simulink model "Neurofeedback_GetConnectivity_IncrementalAvg"  (R2021b)
settings: Solver=ode23tb  StartTime=0.0  StopTime=130  FixedStep=1  RelTol=1e-3
libraries: simulink x6
settings Model: SnapshotBufferSize=100  SnapshotInterval=100  Creator=mariodelossantos  LastModifiedBy=mdls3

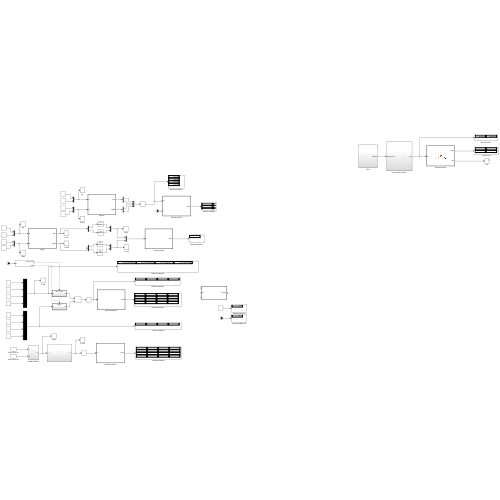
[thumbnail: Simulink's stored preview of the top-level diagram]
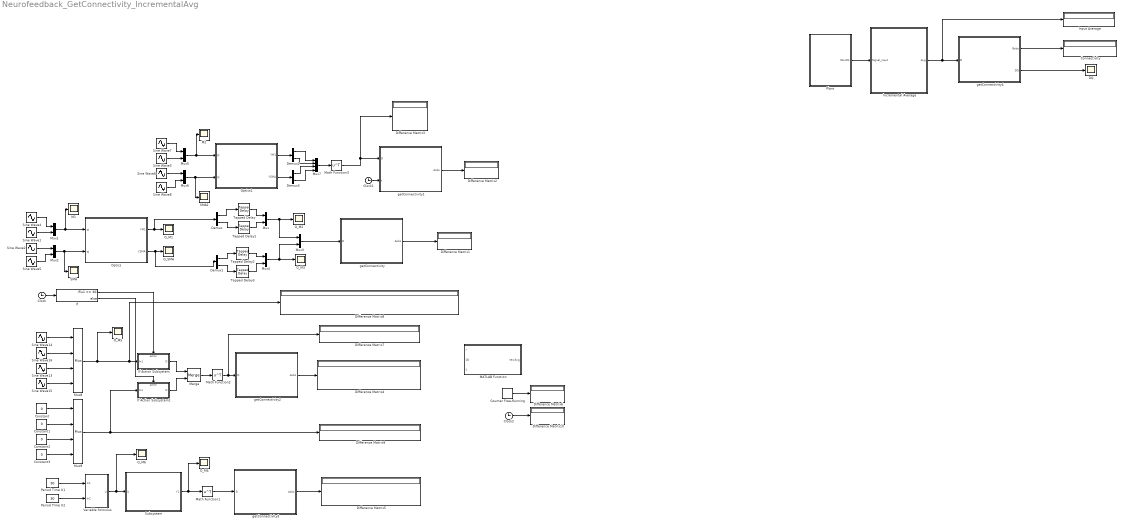
== system Neurofeedback_GetConnectivity_IncrementalAvg ==
  Clock : Clock
  Clock1 : Clock
  Clock2 : Clock
  Connectivity : Display
  Constant{,1..3} (4 alike) : Constant  Value=0
  Counter Free-Running : simulink/Sources/Counter Free-Running  NumBits=16  tsamp=-1
  DQ : Scope
  Demux{,1..3} (4 alike) : Demux  Outputs=2
  Difference Matrix{1..10} (10 alike) : Display
  If : If  IfExpression=u1 == 30
  If Action Subsystem : Subsystem  TreatAsAtomicUnit=on
  If Action Subsystem1 : Subsystem  TreatAsAtomicUnit=on
  Incremental Average : Subsystem
  "Input Average " : Display
  M1 : Scope
  M2 : Scope
  MATLAB Function : MATLAB Function  TreatAsAtomicUnit=on
  Math Function1 : Math  Operator=transpose  SaturateOnIntegerOverflow=on
  Math Function2 : Math  Operator=transpose  SaturateOnIntegerOverflow=on
  Math Function3 : Math  Operator=transpose  SaturateOnIntegerOverflow=on
  Merge : Merge  InitialOutput=[0 0 0 0]
  Mux{,1..6} (7 alike) : Mux  Inputs=2
  Mux7 : Mux
  Mux8 : Mux
  Mux9 : Mux
  O_M{1..6} (6 alike) : Scope
  O_SMA : Scope
  Optics : MATLAB Function  TreatAsAtomicUnit=on
  Optics1 : MATLAB Function  TreatAsAtomicUnit=on
  Period Time U1 : Constant  Value=30
  Period Time U2 : Constant  Value=30
  Plant : Subsystem
  SMA : Scope
  SMA1 : Scope
  Sine Wave1 : Sin  Amplitude=1.2  Frequency=0.8  SampleTime=0
  Sine Wave13 : Sin  Amplitude=0.8  Frequency=0.6  SampleTime=0
  Sine Wave14 : Sin  Frequency=0.9  SampleTime=0
  Sine Wave15 : Sin  Frequency=0.4  SampleTime=0
  Sine Wave16 : Sin  Amplitude=1.2  Frequency=0.8  SampleTime=0
  Sine Wave2 : Sin  Amplitude=0.8  Frequency=0.8  SampleTime=0
  Sine Wave3 : Sin  Amplitude=1.2  Frequency=0.8  SampleTime=0
  Sine Wave{4..5,7..8} (4 alike) : Sin  Frequency=0.8  SampleTime=0
  Sine Wave6 : Sin  Amplitude=0.8  Frequency=0.8  SampleTime=0
  Subsystem : Subsystem
  Tapped Delay{,1..3} (4 alike) : simulink/Discrete/Tapped Delay  vinit=0.0  samptime=-1  NumDelays=29  DelayOrder=Oldest  includeCurrent=on
  Variable Stimulus : Subsystem
  getConnectivity : MATLAB Function  TreatAsAtomicUnit=on  SystemSampleTime=0
  getConnectivity1 : MATLAB Function  TreatAsAtomicUnit=on  SystemSampleTime=0
  getConnectivity2 : MATLAB Function  TreatAsAtomicUnit=on  SystemSampleTime=0
  getConnectivity3 : MATLAB Function  TreatAsAtomicUnit=on  SystemSampleTime=0
  getConnectivity4 : MATLAB Function  TreatAsAtomicUnit=on  SystemSampleTime=0
  wires:
  getConnectivity/1(Aobs) -> Difference Matrix1/1
  Sine Wave4/1 -> Mux1/1
  Sine Wave5/1 -> Mux2/2
  Sine Wave1/1 -> Mux1/2
  Sine Wave2/1 -> Mux2/1
  Optics/1(YM1) -> O_M1/1, Demux/1
  Optics/2(YSMA) -> Demux1/1, O_SMA/1
  Mux2/1 -> SMA/1, Optics/2(qj)
  Mux1/1 -> M1/1, Optics/1(pj)
  Demux/1 -> Tapped Delay/1
  Demux/2 -> Tapped Delay1/1
  Tapped Delay/1 -> Mux/1
  Tapped Delay1/1 -> Mux/2
  Mux/1 -> O_M2/1, Mux3/1
  Mux3/1 -> getConnectivity/1(D)
  Mux4/1 -> O_M3/1, Mux3/2
  Clock/1 -> If/1
  If/1 -> If Action Subsystem/Action
  Tapped Delay2/1 -> Mux4/1
  Demux1/1 -> Tapped Delay2/1
  Demux1/2 -> Tapped Delay3/1
  Tapped Delay3/1 -> Mux4/2
  If/2 -> If Action Subsystem1/Action
  If Action Subsystem/1(D) -> Merge/1
  If Action Subsystem1/1(D) -> Merge/2
  Demux3/1 -> Mux7/3
  Clock1/1 -> getConnectivity1/2(t)
  Demux3/2 -> Mux7/4
  Mux6/1 -> SMA1/1, Optics1/2(qj)
  Sine Wave8/1 -> Mux6/2
  Demux2/1 -> Mux7/1
  Optics1/2(YSMA) -> Demux3/1
  Sine Wave7/1 -> Mux5/1
  Mux5/1 -> M2/1, Optics1/1(pj)
  Optics1/1(YM1) -> Demux2/1
  Sine Wave6/1 -> Mux6/1
  Sine Wave3/1 -> Mux5/2
  Demux2/2 -> Mux7/2
  getConnectivity1/1(Aobs) -> Difference Matrix2/1
  getConnectivity2/1(Aobs) -> Difference Matrix4/1
  getConnectivity3/1(Aobs) -> Difference Matrix5/1
  Merge/1 -> Math Function2/1
  Math Function1/1 -> getConnectivity3/1(D)
  Mux8/1 -> O_M5/1, Difference Matrix8/1, If Action Subsystem/1(In1)
  Sine Wave13/1 -> Mux8/3
  Sine Wave16/1 -> Mux8/2
  Sine Wave15/1 -> Mux8/4
  Sine Wave14/1 -> Mux8/1
  Mux9/1 -> If Action Subsystem1/1(In1), Difference Matrix9/1
  Constant/1 -> Mux9/1
  Constant1/1 -> Mux9/2
  Constant2/1 -> Mux9/3
  Constant3/1 -> Mux9/4
  Math Function2/1 -> getConnectivity2/1(D), Difference Matrix7/1
  Subsystem/1(Y1) -> O_M4/1, Math Function1/1
  Period Time U1/1 -> Variable Stimulus/1(In1)
  Period Time U2/1 -> Variable Stimulus/2(In2)
  Variable Stimulus/1(U) -> O_M6/1, Subsystem/1(U)
  Mux7/1 -> Math Function3/1
  Math Function3/1 -> Difference Matrix3/1, getConnectivity1/1(D)
  Counter Free-Running/1 -> Difference Matrix6/1
  Clock2/1 -> Difference Matrix10/1
  getConnectivity4/1(Bobs) -> Connectivity/1
  Incremental Average/1(Avg) -> getConnectivity4/1(D), "Input Average "/1
  getConnectivity4/2(DQ) -> DQ/1
  Plant/1(DH-DQ) -> Incremental Average/1(Signal_input)

== system Neurofeedback_GetConnectivity_IncrementalAvg/If Action Subsystem ==
  In1 : Inport
  Action Port : ActionPort  ActionPortLabel=if(u1 == 30)
  D : Outport
  wires:
  In1/1 -> D/1

== system Neurofeedback_GetConnectivity_IncrementalAvg/If Action Subsystem1 ==
  In1 : Inport
  Action Port : ActionPort  ActionPortLabel=else
  D : Outport
  wires:
  In1/1 -> D/1

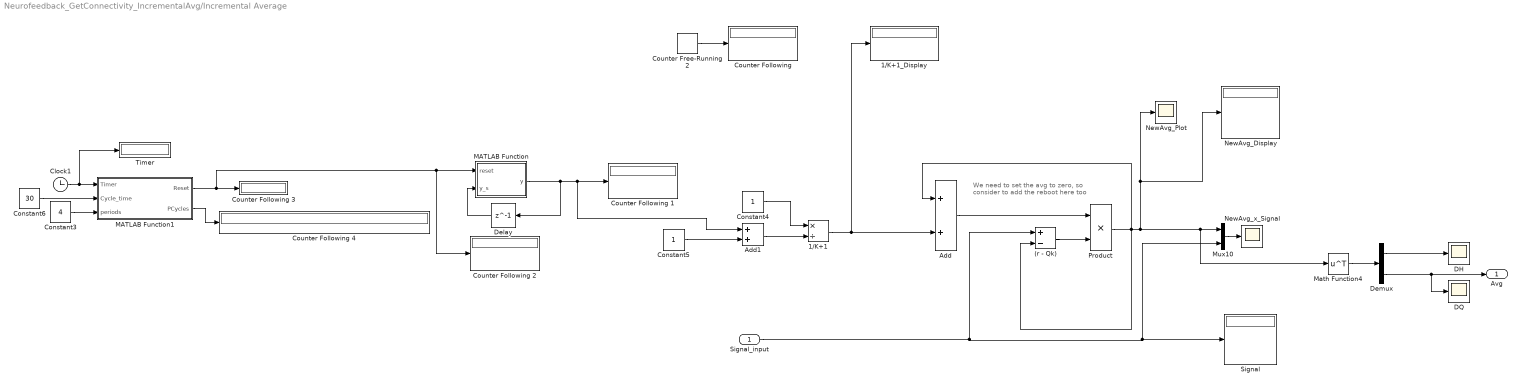
== system Neurofeedback_GetConnectivity_IncrementalAvg/Incremental Average ==
  note: We need to set the avg to zero, so consider to add the reboot here too
  Signal_input : Inport
  (r - Qk) : Sum  Inputs=+-
  1/K+1 : Product  Inputs=*/
  1/K+1_Display : Display
  Add : Sum
  Add1 : Sum
  Clock1 : Clock
  Constant3 : Constant  Value=4
  Constant4 : Constant
  Constant5 : Constant
  Constant6 : Constant  Value=30
  Counter Free-Running2 : simulink/Sources/Counter Free-Running  NumBits=16  tsamp=-1
  Counter Following {,1..4} (5 alike) : Display
  DH : Scope
  DQ : Scope
  Delay : Delay  DelayLength=1  InitialCondition=0
  Demux : Demux  Outputs=2
  MATLAB Function : MATLAB Function  TreatAsAtomicUnit=on
  MATLAB Function1 : MATLAB Function  TreatAsAtomicUnit=on
  Math Function4 : Math  Operator=transpose  SaturateOnIntegerOverflow=on
  Mux10 : Mux  Inputs=2
  NewAvg_Display : Display
  NewAvg_Plot : Scope
  NewAvg_x_Signal : Scope
  Product : Product
  Signal : Display
  Timer : Display
  Avg : Outport
  wires:
  (r - Qk)/1 -> Product/2
  Signal_input/1 -> Signal/1, Mux10/2, (r - Qk)/1
  Add/1 -> Product/1
  Mux10/1 -> NewAvg_x_Signal/1
  Product/1 -> Add/1, (r - Qk)/2, NewAvg_Plot/1, NewAvg_Display/1, Math Function4/1, Mux10/1
  Math Function4/1 -> Demux/1
  Demux/2 -> Avg/1, DQ/1
  Demux/1 -> DH/1
  Constant4/1 -> 1/K+1/1
  Counter Free-Running2/1 -> "Counter Following "/1
  Constant5/1 -> Add1/2
  Add1/1 -> 1/K+1/2
  1/K+1/1 -> 1/K+1_Display/1, Add/2
  MATLAB Function/1(y) -> Add1/1, Counter Following 1/1, Delay/1
  Delay/1 -> MATLAB Function/2(y_s)
  MATLAB Function1/1(Reset) -> Counter Following 2/1, MATLAB Function/1(reset), Counter Following 3/1
  MATLAB Function1/2(PCycles) -> Counter Following 4/1
  Constant6/1 -> MATLAB Function1/2(Cycle_time)
  Constant3/1 -> MATLAB Function1/3(periods)
  Clock1/1 -> MATLAB Function1/1(Timer), Timer/1

== system Neurofeedback_GetConnectivity_IncrementalAvg/Plant ==
  Human Agent : Subsystem
  Period Time U3 : Constant  Value=30
  Period Time U4 : Constant  Value=30
  Stimulus : Scope
  Variable Stimulus1 : Subsystem
  fNIRS : Scope
  DH-DQ : Outport
  wires:
  Human Agent/1(fNIRS) -> fNIRS/1
  Period Time U3/1 -> Variable Stimulus1/1(In1)
  Period Time U4/1 -> Variable Stimulus1/2(In2)
  Human Agent/2(DH-DQ) -> DH-DQ/1
  Variable Stimulus1/1(U) -> Stimulus/1, Human Agent/1(Stimulus)

== system Neurofeedback_GetConnectivity_IncrementalAvg/Subsystem ==
  U : Inport
  Deltas-Hemo1 : Subsystem
  Hemodynamics1 : Subsystem
  Neurodynamics1 : Subsystem
  Optics2 : Subsystem
  Z : Scope
  y1 : Scope
  Y1 : Outport
  wires:
  Deltas-Hemo1/1(DH) -> Optics2/1(DH)
  U/1 -> Neurodynamics1/1(U)
  Neurodynamics1/1(Z) -> Z/1, Hemodynamics1/1(Zj)  "Zj"
  Deltas-Hemo1/2(DQ) -> Optics2/2(DQ)
  Optics2/1(Y1) -> y1/1, Y1/1
  Hemodynamics1/1(Pj) -> Deltas-Hemo1/1(pj)
  Hemodynamics1/2(qj) -> Deltas-Hemo1/2(qj)

== system Neurofeedback_GetConnectivity_IncrementalAvg/Variable Stimulus ==
  In1 : Inport
  In2 : Inport  Port=2
  Duty-Cycle-U1 : Constant  Value=0.16667  OutMin=[0]  OutMax=[0.8]
  Duty-Cycle-U2 : Constant  Value=0.16667  OutMin=[0]  OutMax=[0.8]
  Mux : Mux  Inputs=2
  Variable Pulse Generator1 : VariablePulseGenerator  RunAtFixedTimeIntervals=on
  Variable Pulse Generator2 : VariablePulseGenerator  RunAtFixedTimeIntervals=on
  U : Outport
  wires:
  In2/1 -> Variable Pulse Generator1/2
  Mux/1 -> U/1
  Variable Pulse Generator1/1 -> Mux/2
  Duty-Cycle-U2/1 -> Variable Pulse Generator1/1
  In1/1 -> Variable Pulse Generator2/2
  Duty-Cycle-U1/1 -> Variable Pulse Generator2/1
  Variable Pulse Generator2/1 -> Mux/1

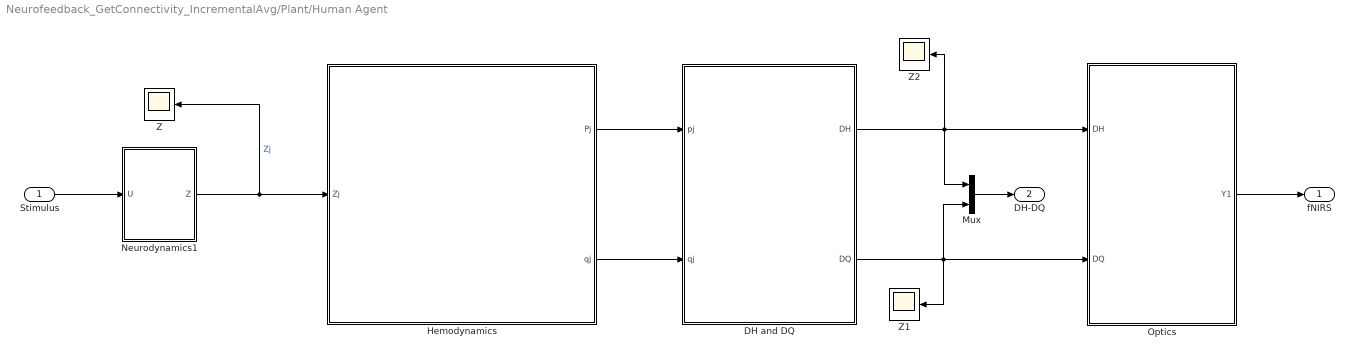
== system Neurofeedback_GetConnectivity_IncrementalAvg/Plant/Human Agent ==
  Stimulus : Inport
  DH and DQ : Subsystem
  Hemodynamics : Subsystem
  Mux : Mux  Inputs=2
  Neurodynamics1 : Subsystem
  Optics : Subsystem
  Z : Scope
  Z1 : Scope
  Z2 : Scope
  fNIRS : Outport
  DH-DQ : Outport  Port=2
  wires:
  Hemodynamics/1(Pj) -> DH and DQ/1(pj)
  Hemodynamics/2(qj) -> DH and DQ/2(qj)
  Neurodynamics1/1(Z) -> Z/1, Hemodynamics/1(Zj)  "Zj"
  Stimulus/1 -> Neurodynamics1/1(U)
  DH and DQ/1(DH) -> Z2/1, Mux/1, Optics/1(DH)
  DH and DQ/2(DQ) -> Z1/1, Mux/2, Optics/2(DQ)
  Optics/1(Y1) -> fNIRS/1
  Mux/1 -> DH-DQ/1

== system Neurofeedback_GetConnectivity_IncrementalAvg/Plant/Variable Stimulus1 ==
  In1 : Inport
  In2 : Inport  Port=2
  Duty-Cycle-U1 : Constant  Value=0.16667  OutMin=[0]  OutMax=[0.8]
  Duty-Cycle-U2 : Constant  Value=0.16667  OutMin=[0]  OutMax=[0.8]
  Mux : Mux  Inputs=2
  Variable Pulse Generator1 : VariablePulseGenerator  RunAtFixedTimeIntervals=on  SampleTime=1/100
  Variable Pulse Generator2 : VariablePulseGenerator  RunAtFixedTimeIntervals=on  SampleTime=1/100
  U : Outport
  wires:
  In2/1 -> Variable Pulse Generator1/2
  Mux/1 -> U/1
  Variable Pulse Generator1/1 -> Mux/2
  Duty-Cycle-U2/1 -> Variable Pulse Generator1/1
  In1/1 -> Variable Pulse Generator2/2
  Duty-Cycle-U1/1 -> Variable Pulse Generator2/1
  Variable Pulse Generator2/1 -> Mux/1

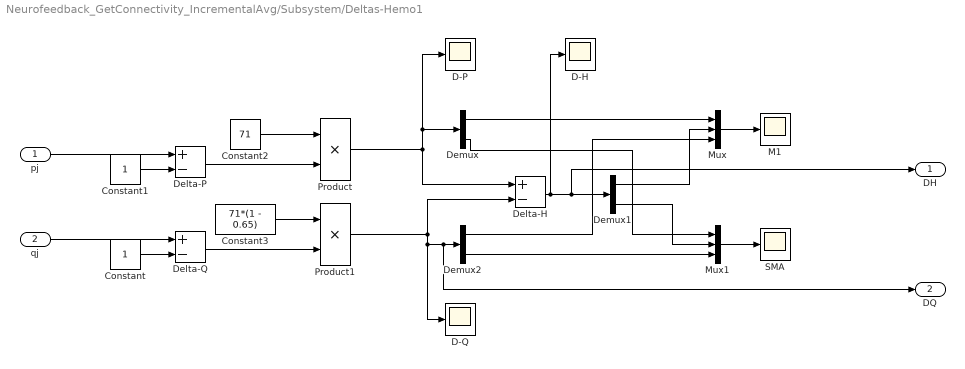
== system Neurofeedback_GetConnectivity_IncrementalAvg/Subsystem/Deltas-Hemo1 ==
  pj : Inport
  qj : Inport  Port=2
  Constant : Constant
  Constant1 : Constant
  Constant2 : Constant  Value=71
  Constant3 : Constant  Value=71*(1 - 0.65)
  D-H : Scope
  D-P : Scope
  D-Q : Scope
  Delta-H : Sum  Inputs=+-
  Delta-P : Sum  Inputs=+-
  Delta-Q : Sum  Inputs=+-
  Demux : Demux  Outputs=2
  Demux1 : Demux  Outputs=2
  Demux2 : Demux  Outputs=2
  M1 : Scope
  Mux : Mux  Inputs=3
  Mux1 : Mux  Inputs=3
  Product : Product
  Product1 : Product
  SMA : Scope
  DH : Outport
  DQ : Outport  Port=2
  wires:
  Constant2/1 -> Product/1
  Delta-Q/1 -> Product1/2
  Constant3/1 -> Product1/1
  Demux2/2 -> Mux1/3
  pj/1 -> Delta-P/1
  Mux1/1 -> SMA/1
  Demux/2 -> Mux1/1
  Mux/1 -> M1/1
  Constant/1 -> Delta-Q/2
  Delta-P/1 -> Product/2
  Product1/1 -> DQ/1, Demux2/1, D-Q/1, Delta-H/2
  qj/1 -> Delta-Q/1
  Demux/1 -> Mux/1
  Delta-H/1 -> DH/1, Demux1/1, D-H/1
  Demux1/1 -> Mux/2
  Demux1/2 -> Mux1/2
  Product/1 -> Demux/1, D-P/1, Delta-H/1
  Demux2/1 -> Mux/3
  Constant1/1 -> Delta-P/2

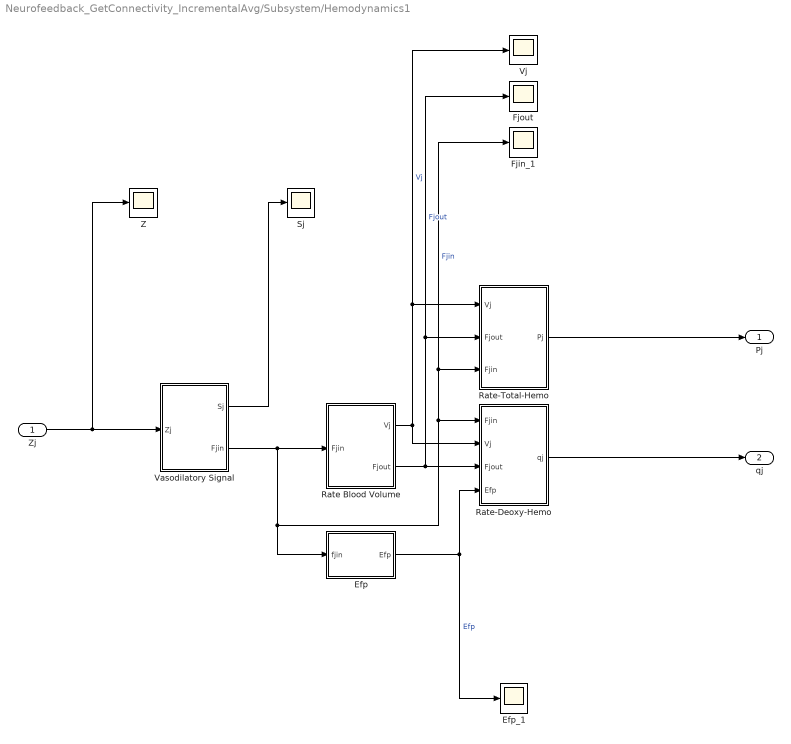
== system Neurofeedback_GetConnectivity_IncrementalAvg/Subsystem/Hemodynamics1 ==
  Zj : Inport
  Efp : MATLAB Function  TreatAsAtomicUnit=on
  Efp_1 : Scope
  Fjin_1 : Scope
  Fjout : Scope
  Rate Blood Volume : Subsystem
  Rate-Deoxy-Hemo : Subsystem
  Rate-Total-Hemo : Subsystem
  Sj : Scope
  Vasodilatory Signal : Subsystem
  Vj : Scope
  Z : Scope
  Pj : Outport
  qj : Outport  Port=2
  wires:
  Rate-Deoxy-Hemo/1(qj) -> qj/1
  Zj/1 -> Vasodilatory Signal/1(Zj), Z/1
  Vasodilatory Signal/1(Sj) -> Sj/1
  Rate Blood Volume/2(Fjout) -> Fjout/1, Rate-Total-Hemo/2(Fjout), Rate-Deoxy-Hemo/3(Fjout)  "Fjout"
  Rate Blood Volume/1(Vj) -> Vj/1, Rate-Total-Hemo/1(Vj), Rate-Deoxy-Hemo/2(Vj)  "Vj"
  Rate-Total-Hemo/1(Pj) -> Pj/1
  Efp/1(Efp) -> Rate-Deoxy-Hemo/4(Efp), Efp_1/1  "Efp"
  Vasodilatory Signal/2(Fjin) -> Efp/1(fjin), Fjin_1/1, Rate-Total-Hemo/3(Fjin), Rate-Deoxy-Hemo/1(Fjin), Rate Blood Volume/1(Fjin)  "Fjin"

== system Neurofeedback_GetConnectivity_IncrementalAvg/Subsystem/Neurodynamics1 ==
  U : Inport
  C : Gain  Gain=[0.08 0;0.06 0]  Multiplication=Matrix(K*u)
  Integrator : Integrator
  Jt : MATLAB Function  TreatAsAtomicUnit=on
  Sum : Sum  Inputs=|++
  Z : Outport
  wires:
  Integrator/1 -> Z/1, Jt/1(Zt)
  C/1 -> Sum/1
  Jt/1(Jt) -> Sum/2
  U/1 -> C/1, Jt/2(U)
  Sum/1 -> Integrator/1

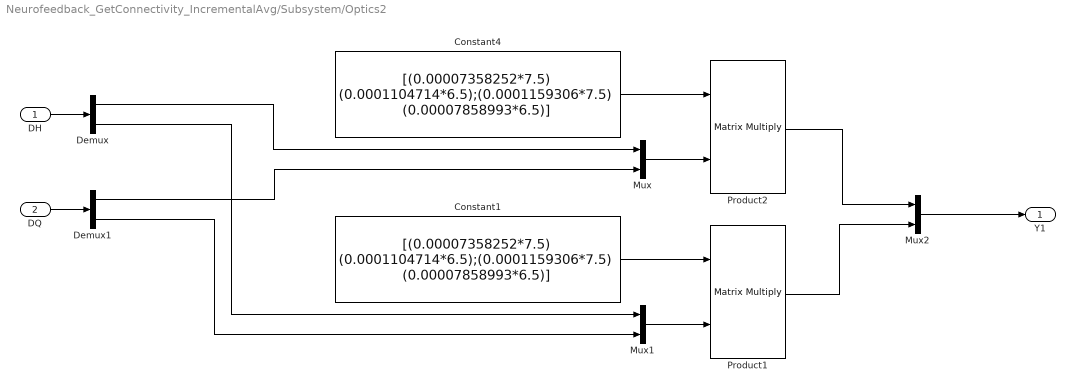
== system Neurofeedback_GetConnectivity_IncrementalAvg/Subsystem/Optics2 ==
  DH : Inport
  DQ : Inport  Port=2
  Constant1 : Constant  Value=[(0.00007358252*7.5) (0.0001104714*6.5);(0.0001159306*7.5) (0.00007858993*6.5)]
  Constant4 : Constant  Value=[(0.00007358252*7.5) (0.0001104714*6.5);(0.0001159306*7.5) (0.00007858993*6.5)]
  Demux : Demux  Outputs=2
  Demux1 : Demux  Outputs=2
  Mux : Mux  Inputs=2
  Mux1 : Mux  Inputs=2
  Mux2 : Mux  Inputs=2
  Product1 : Product  Multiplication=Matrix(*)
  Product2 : Product  Multiplication=Matrix(*)
  Y1 : Outport
  wires:
  Mux/1 -> Product2/2
  Product2/1 -> Mux2/1
  Mux1/1 -> Product1/2
  Product1/1 -> Mux2/2
  Constant1/1 -> Product1/1
  DH/1 -> Demux/1
  Demux/1 -> Mux/1
  Demux/2 -> Mux1/1
  DQ/1 -> Demux1/1
  Constant4/1 -> Product2/1
  Demux1/1 -> Mux/2
  Demux1/2 -> Mux1/2
  Mux2/1 -> Y1/1

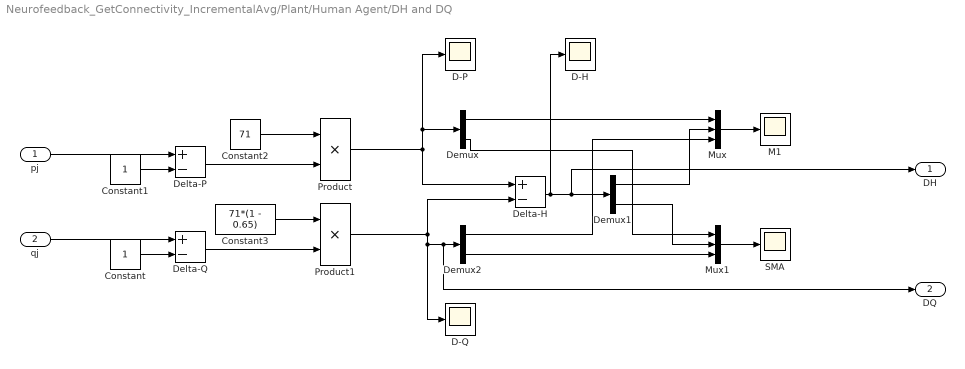
== system Neurofeedback_GetConnectivity_IncrementalAvg/Plant/Human Agent/DH and DQ ==
  pj : Inport
  qj : Inport  Port=2
  Constant : Constant
  Constant1 : Constant
  Constant2 : Constant  Value=71
  Constant3 : Constant  Value=71*(1 - 0.65)
  D-H : Scope
  D-P : Scope
  D-Q : Scope
  Delta-H : Sum  Inputs=+-
  Delta-P : Sum  Inputs=+-
  Delta-Q : Sum  Inputs=+-
  Demux : Demux  Outputs=2
  Demux1 : Demux  Outputs=2
  Demux2 : Demux  Outputs=2
  M1 : Scope
  Mux : Mux  Inputs=3
  Mux1 : Mux  Inputs=3
  Product : Product
  Product1 : Product
  SMA : Scope
  DH : Outport
  DQ : Outport  Port=2
  wires:
  Constant2/1 -> Product/1
  Delta-Q/1 -> Product1/2
  Constant3/1 -> Product1/1
  Demux2/2 -> Mux1/3
  pj/1 -> Delta-P/1
  Mux1/1 -> SMA/1
  Demux/2 -> Mux1/1
  Mux/1 -> M1/1
  Constant/1 -> Delta-Q/2
  Delta-P/1 -> Product/2
  Product1/1 -> DQ/1, Demux2/1, D-Q/1, Delta-H/2
  qj/1 -> Delta-Q/1
  Demux/1 -> Mux/1
  Delta-H/1 -> DH/1, Demux1/1, D-H/1
  Demux1/1 -> Mux/2
  Demux1/2 -> Mux1/2
  Product/1 -> Demux/1, D-P/1, Delta-H/1
  Demux2/1 -> Mux/3
  Constant1/1 -> Delta-P/2

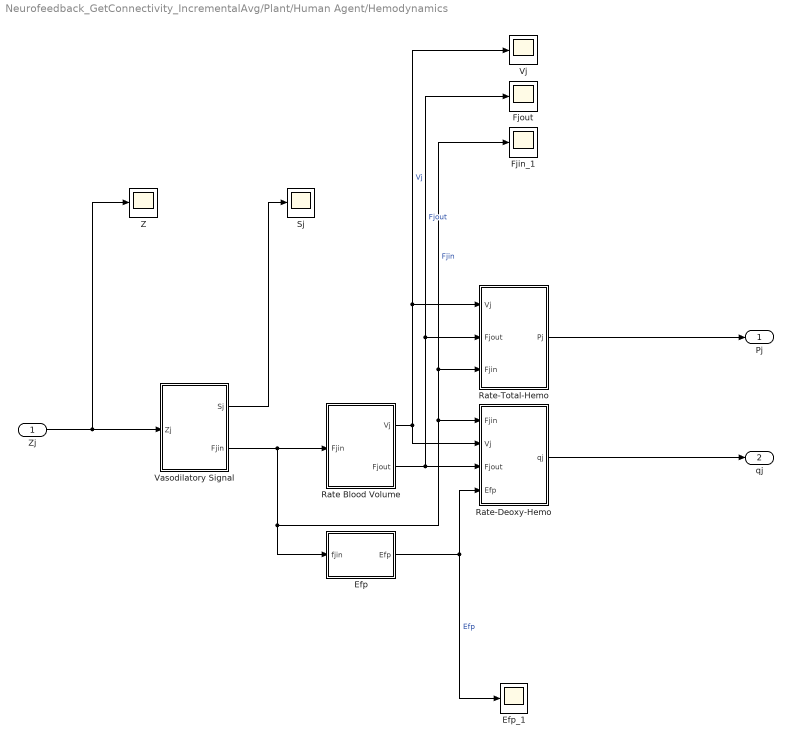
== system Neurofeedback_GetConnectivity_IncrementalAvg/Plant/Human Agent/Hemodynamics ==
  Zj : Inport
  Efp : MATLAB Function  TreatAsAtomicUnit=on
  Efp_1 : Scope
  Fjin_1 : Scope
  Fjout : Scope
  Rate Blood Volume : Subsystem
  Rate-Deoxy-Hemo : Subsystem
  Rate-Total-Hemo : Subsystem
  Sj : Scope
  Vasodilatory Signal : Subsystem
  Vj : Scope
  Z : Scope
  Pj : Outport
  qj : Outport  Port=2
  wires:
  Rate-Deoxy-Hemo/1(qj) -> qj/1
  Zj/1 -> Vasodilatory Signal/1(Zj), Z/1
  Vasodilatory Signal/1(Sj) -> Sj/1
  Rate Blood Volume/2(Fjout) -> Fjout/1, Rate-Total-Hemo/2(Fjout), Rate-Deoxy-Hemo/3(Fjout)  "Fjout"
  Rate Blood Volume/1(Vj) -> Vj/1, Rate-Total-Hemo/1(Vj), Rate-Deoxy-Hemo/2(Vj)  "Vj"
  Rate-Total-Hemo/1(Pj) -> Pj/1
  Efp/1(Efp) -> Rate-Deoxy-Hemo/4(Efp), Efp_1/1  "Efp"
  Vasodilatory Signal/2(Fjin) -> Efp/1(fjin), Fjin_1/1, Rate-Total-Hemo/3(Fjin), Rate-Deoxy-Hemo/1(Fjin), Rate Blood Volume/1(Fjin)  "Fjin"

== system Neurofeedback_GetConnectivity_IncrementalAvg/Plant/Human Agent/Neurodynamics1 ==
  U : Inport
  C : Gain  Gain=[0.08 0;0.06 0]  Multiplication=Matrix(K*u)
  Integrator : Integrator
  Jt : MATLAB Function  TreatAsAtomicUnit=on
  Sum : Sum  Inputs=|++
  Z : Outport
  wires:
  Integrator/1 -> Z/1, Jt/1(Zt)
  C/1 -> Sum/1
  Jt/1(Jt) -> Sum/2
  U/1 -> C/1, Jt/2(U)
  Sum/1 -> Integrator/1

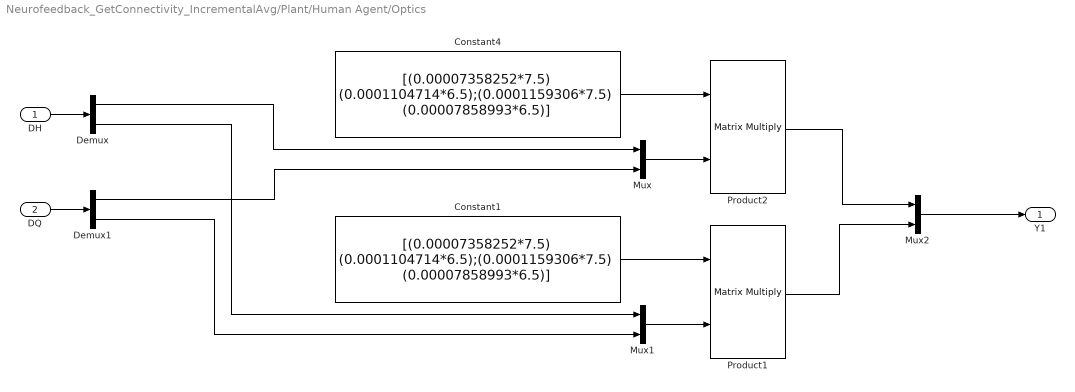
== system Neurofeedback_GetConnectivity_IncrementalAvg/Plant/Human Agent/Optics ==
  DH : Inport
  DQ : Inport  Port=2
  Constant1 : Constant  Value=[(0.00007358252*7.5) (0.0001104714*6.5);(0.0001159306*7.5) (0.00007858993*6.5)]
  Constant4 : Constant  Value=[(0.00007358252*7.5) (0.0001104714*6.5);(0.0001159306*7.5) (0.00007858993*6.5)]
  Demux : Demux  Outputs=2
  Demux1 : Demux  Outputs=2
  Mux : Mux  Inputs=2
  Mux1 : Mux  Inputs=2
  Mux2 : Mux  Inputs=2
  Product1 : Product  Multiplication=Matrix(*)
  Product2 : Product  Multiplication=Matrix(*)
  Y1 : Outport
  wires:
  Mux/1 -> Product2/2
  Product2/1 -> Mux2/1
  Mux1/1 -> Product1/2
  Product1/1 -> Mux2/2
  Constant1/1 -> Product1/1
  DH/1 -> Demux/1
  Demux/1 -> Mux/1
  Demux/2 -> Mux1/1
  DQ/1 -> Demux1/1
  Constant4/1 -> Product2/1
  Demux1/1 -> Mux/2
  Demux1/2 -> Mux1/2
  Mux2/1 -> Y1/1

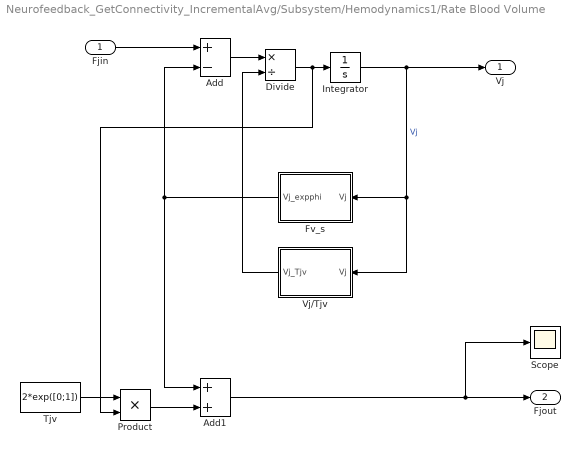
== system Neurofeedback_GetConnectivity_IncrementalAvg/Subsystem/Hemodynamics1/Rate Blood Volume ==
  Fjin : Inport
  Add : Sum  Inputs=+-
  Add1 : Sum
  Divide : Product  Inputs=*/
  Fv_s : MATLAB Function  TreatAsAtomicUnit=on
  Integrator : Integrator  InitialCondition=exp([0;0])
  Product : Product
  Scope : Scope
  Tjv : Constant  Value=2*exp([0;1])
  Vj/Tjv : MATLAB Function  TreatAsAtomicUnit=on
  Vj : Outport
  Fjout : Outport  Port=2
  wires:
  Fjin/1 -> Add/1
  Integrator/1 -> Vj/1, Vj/Tjv/1(Vj), Fv_s/1(Vj)  "Vj"
  Divide/1 -> Product/2, Integrator/1
  Fv_s/1(Vj_expphi) -> Add/2, Add1/1
  Add/1 -> Divide/1
  Vj/Tjv/1(Vj_Tjv) -> Divide/2
  Product/1 -> Add1/2
  Tjv/1 -> Product/1
  Add1/1 -> Scope/1, Fjout/1

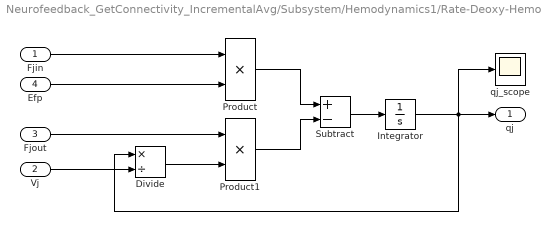
== system Neurofeedback_GetConnectivity_IncrementalAvg/Subsystem/Hemodynamics1/Rate-Deoxy-Hemo ==
  Fjin : Inport
  Vj : Inport  Port=2
  Fjout : Inport  Port=3
  Efp : Inport  Port=4
  Divide : Product  Inputs=*/
  Integrator : Integrator  InitialCondition=exp([0;0])
  Product : Product
  Product1 : Product
  Subtract : Sum  Inputs=+-
  qj_scope : Scope
  qj : Outport
  wires:
  Efp/1 -> Product/2
  Divide/1 -> Product1/2
  Subtract/1 -> Integrator/1
  Integrator/1 -> qj/1, Divide/1, qj_scope/1
  Vj/1 -> Divide/2
  Product1/1 -> Subtract/2
  Fjin/1 -> Product/1
  Fjout/1 -> Product1/1
  Product/1 -> Subtract/1

== system Neurofeedback_GetConnectivity_IncrementalAvg/Subsystem/Hemodynamics1/Rate-Total-Hemo ==
  Vj : Inport
  Fjout : Inport  Port=2
  Fjin : Inport  Port=3
  Divide : Product  Inputs=*/
  Integrator : Integrator  InitialCondition=exp([0;0])
  Product : Product
  Subtract : Sum  Inputs=+-
  pj : Scope
  Pj : Outport
  wires:
  Fjout/1 -> Subtract/2
  Product/1 -> Integrator/1
  Vj/1 -> Divide/2
  Subtract/1 -> Product/1
  Fjin/1 -> Subtract/1
  Divide/1 -> Product/2
  Integrator/1 -> Pj/1, pj/1, Divide/1

== system Neurofeedback_GetConnectivity_IncrementalAvg/Subsystem/Hemodynamics1/Vasodilatory Signal ==
  Zj : Inport
  Add : Sum  Inputs=+--
  Add1 : Sum  Inputs=+-
  Constant1 : Constant
  Integrator : Integrator
  Integrator1 : Integrator  InitialCondition=exp([0;0])
  K : Gain  Gain=0.64*exp([0;0.05])
  Scope1 : Scope
  Yj : Gain  Gain=0.32*exp([0;0.05])
  Sj : Outport
  Fjin : Outport  Port=2
  wires:
  Add1/1 -> Yj/1
  K/1 -> Add/2  "Kj*Sj"
  Constant1/1 -> Add1/2
  Zj/1 -> Add/1
  Integrator1/1 -> Fjin/1, Scope1/1, Add1/1
  Integrator/1 -> Sj/1, K/1, Integrator1/1
  Add/1 -> Integrator/1
  Yj/1 -> Add/3  "Yj(Fjin - 1)"

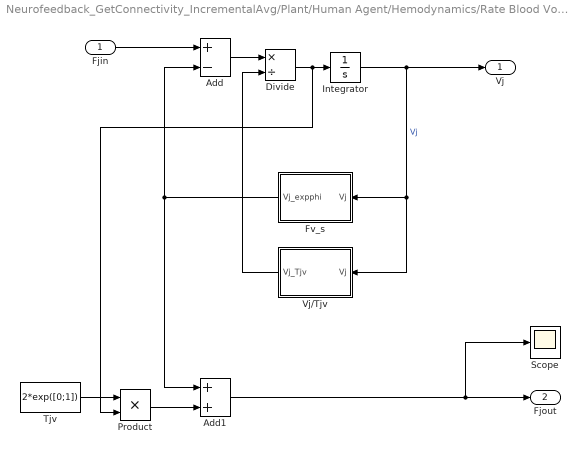
== system Neurofeedback_GetConnectivity_IncrementalAvg/Plant/Human Agent/Hemodynamics/Rate Blood Volume ==
  Fjin : Inport
  Add : Sum  Inputs=+-
  Add1 : Sum
  Divide : Product  Inputs=*/
  Fv_s : MATLAB Function  TreatAsAtomicUnit=on
  Integrator : Integrator  InitialCondition=exp([0;0])
  Product : Product
  Scope : Scope
  Tjv : Constant  Value=2*exp([0;1])
  Vj/Tjv : MATLAB Function  TreatAsAtomicUnit=on
  Vj : Outport
  Fjout : Outport  Port=2
  wires:
  Fjin/1 -> Add/1
  Integrator/1 -> Vj/1, Vj/Tjv/1(Vj), Fv_s/1(Vj)  "Vj"
  Divide/1 -> Product/2, Integrator/1
  Fv_s/1(Vj_expphi) -> Add/2, Add1/1
  Add/1 -> Divide/1
  Vj/Tjv/1(Vj_Tjv) -> Divide/2
  Product/1 -> Add1/2
  Tjv/1 -> Product/1
  Add1/1 -> Scope/1, Fjout/1

== system Neurofeedback_GetConnectivity_IncrementalAvg/Plant/Human Agent/Hemodynamics/Rate-Deoxy-Hemo ==
  Fjin : Inport
  Vj : Inport  Port=2
  Fjout : Inport  Port=3
  Efp : Inport  Port=4
  Divide : Product  Inputs=*/
  Integrator : Integrator  InitialCondition=exp([0;0])
  Product : Product
  Product1 : Product
  Subtract : Sum  Inputs=+-
  qj_scope : Scope
  qj : Outport
  wires:
  Efp/1 -> Product/2
  Divide/1 -> Product1/2
  Subtract/1 -> Integrator/1
  Integrator/1 -> qj/1, Divide/1, qj_scope/1
  Vj/1 -> Divide/2
  Product1/1 -> Subtract/2
  Fjin/1 -> Product/1
  Fjout/1 -> Product1/1
  Product/1 -> Subtract/1

== system Neurofeedback_GetConnectivity_IncrementalAvg/Plant/Human Agent/Hemodynamics/Rate-Total-Hemo ==
  Vj : Inport
  Fjout : Inport  Port=2
  Fjin : Inport  Port=3
  Divide : Product  Inputs=*/
  Integrator : Integrator  InitialCondition=exp([0;0])
  Product : Product
  Subtract : Sum  Inputs=+-
  pj : Scope
  Pj : Outport
  wires:
  Fjout/1 -> Subtract/2
  Product/1 -> Integrator/1
  Vj/1 -> Divide/2
  Subtract/1 -> Product/1
  Fjin/1 -> Subtract/1
  Divide/1 -> Product/2
  Integrator/1 -> Pj/1, pj/1, Divide/1

== system Neurofeedback_GetConnectivity_IncrementalAvg/Plant/Human Agent/Hemodynamics/Vasodilatory Signal ==
  Zj : Inport
  Add : Sum  Inputs=+--
  Add1 : Sum  Inputs=+-
  Constant1 : Constant
  Integrator : Integrator
  Integrator1 : Integrator  InitialCondition=exp([0;0])
  K : Gain  Gain=0.64*exp([0;0.05])
  Scope1 : Scope
  Yj : Gain  Gain=0.32*exp([0;0.05])
  Sj : Outport
  Fjin : Outport  Port=2
  wires:
  Add1/1 -> Yj/1
  K/1 -> Add/2  "Kj*Sj"
  Constant1/1 -> Add1/2
  Zj/1 -> Add/1
  Integrator1/1 -> Fjin/1, Scope1/1, Add1/1
  Integrator/1 -> Sj/1, K/1, Integrator1/1
  Add/1 -> Integrator/1
  Yj/1 -> Add/3  "Yj(Fjin - 1)"

== matlab function Neurofeedback_GetConnectivity_IncrementalAvg/Plant/Human Agent/Hemodynamics/Rate Blood Volume/Fv_s ==
  data: Vj input; Vj_expphi output
function Vj_expphi = fcn(Vj)
phi = 0.32;
Vj_expphi = Vj.^(1/phi);

== matlab function Neurofeedback_GetConnectivity_IncrementalAvg/getConnectivity1 ==
  data: D input; Aobs output; t input
function Aobs   = getConnectivity(D,t)
    %A = size(4,300);
    %global A;
    %A(:,t) = D;
    
    rThresh= 0.4; % [0..1] A threshold on the correlation.
    [nSamples, nChannels, nHb]=size(D);
    C = nan(nChannels, nChannels, nHb); %Matrix of channel pairwise correlations;

    %This part of the algorithm is HIGHLY inefficient but it does the job for now
    %but might not be sufficiently fast for "real time" neurofeedback
    if(t==30)
        for iHb = 1:nHb

            for iCh=1:nChannels

                for jCh=iCh:nChannels

                    if iCh == jCh

                     C(iCh,jCh,iHb) = 1;

                   else

                     C(iCh,jCh,iHb) = 0;
                     %corr(D(:,iCh,iHb),D(:,jCh,iHb));

                    end
                end

            end

        end
    end

    %Threshold/Binarize C

    tmp = C > rThresh;

    %Finally "merge" accross Hb species

    Aobs = all(tmp,3); %Apply the AND function across Hb species.

== matlab function Neurofeedback_GetConnectivity_IncrementalAvg/Plant/Human Agent/Hemodynamics/Rate Blood Volume/Vj//Tjv ==
  data: Vj input; Vj_Tjv output
function Vj_Tjv = fcn(Vj)
    Tjv = 2*exp([0;1]);
    Tj = 2*exp([0;0.05]);
Vj_Tjv =(Tj.*Tjv.*Vj);

== matlab function Neurofeedback_GetConnectivity_IncrementalAvg/Plant/Human Agent/Neurodynamics1/Jt ==
  data: Zt input; U input; Jt output
function Jt = fcn(Zt, U)
   A = [-0.16 -0.49;-0.02 -0.33];
   nRegions  = size(A,1);
   M = size(U,1); %nStimuli
   simulationLength = size(U,2);
   B = zeros(2,2,2);
   B1 = [0 0; 0 0]; %There must be a B per stimulus
   B2 = [-0.02 -0.77; 0.33 -1.31];
   B(:,:,1) = B1;
   B(:,:,2) = B2;
      assert(M == size(B,3),...
       'Unexpected number of induced connectivity parameters B.');
   T = zeros(nRegions); %nRegions x nRegions
    for t = 1:simulationLength
           for uu = 1:M % Sum (Uj * Bj)
               tmp = U(uu,t)*B(:,:,uu);
               T = -0.5*exp(T + tmp);  
           end
    end
    SI = diag(A);
    A =  A - diag(exp(SI) + (SI));
Jt = (A*Zt) + (T*Zt);

== matlab function Neurofeedback_GetConnectivity_IncrementalAvg/getConnectivity4 ==
  data: D input; Bobs output; DQ output
function [Bobs, DQ] = getConnectivity(D)

    DQ = [nan;nan];
    DQ(1) = D(1);
    DQ(2) = D(2);

    rThresh= 0.6; % [0..1] A threshold on the correlation.

    [nSamples, nChannels, nHb] = size(D);

    C = nan(nChannels, nChannels, nHb); %Matrix of channel pairwise correlations;

    %This part of the algorithm is HIGHLY inefficient but it does the job for now
    %but might not be sufficiently fast for "real time" neurofeedback

    for iHb = 1:nHb
        for iCh=1:nChannels
            for jCh=iCh:nChannels

                if iCh == jCh

                 C(iCh,jCh,iHb) = 1;

               else

                 C(iCh,jCh,iHb) = xcorr2(D(:,iCh,iHb),D(:,jCh,iHb));

                end
            end

        end

    end

    %Threshold/Binarize C

    tmp = C > rThresh;

    %Finally "merge" accross Hb species

    Bobs = all(tmp,3); %Apply the AND function across Hb species.

== matlab function Neurofeedback_GetConnectivity_IncrementalAvg/Incremental Average/MATLAB Function ==
  data: reset input; y_s input; y output
function y = fcn(reset, y_s)

if reset == 1
    y = 0;
else 
    y = y_s + 1;
end

== matlab function Neurofeedback_GetConnectivity_IncrementalAvg/Incremental Average/MATLAB Function1 ==
  data: Timer input; Reset output; Cycle_time input; periods input; PCycles output
function [Reset, PCycles] = fcn(Timer, Cycle_time, periods)

temp = 0;
PCycles = zeros(4,1);
for i = 1:periods
    PCycles(i) = i * Cycle_time;
    if (Timer >= PCycles(i) && Timer <= PCycles(i)+1)
        temp = 1;
        break
    else
        temp = 0;
    end
end 
Reset = temp;

== matlab function Neurofeedback_GetConnectivity_IncrementalAvg/Optics1 ==
  data: pj input; YM1 output; qj input; YSMA output
function [YM1, YSMA]   = Optics(pj, qj)

    N = [0.65 71 2]; 
    P0 = N(2);
    % baseline dxy-hb concentration 
    base_hbr = N(2) * (1-N(1)); 

    F_P =[(0.00007358252*7.5) (0.0001104714*6.5);(0.0001159306*7.5) (0.00007858993*6.5)];
        % calculate changes in hemoglobin concentration
    dp = (pj - 1)* P0; % total Hb
    dq = (qj-1)*base_hbr; % dxy-Hb
    dh = dp - dq; % oxy-Hb
   
    dhq_r1 = [dh(1);dq(1)]; %DH y DQ de M1
    dhq_r2 = [dh(2);dq(2)]; %DH y DQ de SMA
            
YM1 = F_P * dhq_r1;
YSMA = F_P * dhq_r2 ;

== matlab function Neurofeedback_GetConnectivity_IncrementalAvg/Optics ==
  data: pj input; YM1 output; qj input; YSMA output
function [YM1, YSMA]   = Optics(pj, qj)

    N = [0.65 71 2]; 
    P0 = N(2);
    % baseline dxy-hb concentration 
    base_hbr = N(2) * (1-N(1)); 

    F_P =[(0.00007358252*7.5) (0.0001104714*6.5);(0.0001159306*7.5) (0.00007858993*6.5)];
        % calculate changes in hemoglobin concentration
    dp = (pj - 1)* P0; % total Hb
    dq = (qj-1)*base_hbr; % dxy-Hb
    dh = dp - dq; % oxy-Hb
   
    dhq_r1 = [dh(1);dq(1)]; %DH y DQ de M1
    dhq_r2 = [dh(2);dq(2)]; %DH y DQ de SMA
            
YM1 = F_P * dhq_r1;
YSMA = F_P * dhq_r2 ;

== matlab function Neurofeedback_GetConnectivity_IncrementalAvg/getConnectivity2 ==
  data: D input; Aobs output
function Aobs   = getConnectivity(D)

 
    rThresh= 0.6; % [0..1] A threshold on the correlation.

    [nSamples, nChannels, nHb]=size(D);

    C = nan(nChannels, nChannels, nHb); %Matrix of channel pairwise correlations;

    %This part of the algorithm is HIGHLY inefficient but it does the job for now
    %but might not be sufficiently fast for "real time" neurofeedback

    for iHb = 1:nHb
        for iCh=1:nChannels
            for jCh=iCh:nChannels

                if iCh == jCh

                 C(iCh,jCh,iHb) = 1;

               else

                 C(iCh,jCh,iHb) = 0;
                 %corr(D(:,iCh,iHb),D(:,jCh,iHb));

                end
            end

        end

    end

    %Threshold/Binarize C

    tmp = C > rThresh;

    %Finally "merge" accross Hb species

    Aobs = all(tmp,3); %Apply the AND function across Hb species.

== matlab function Neurofeedback_GetConnectivity_IncrementalAvg/getConnectivity ==
  data: D input; Aobs output
function Aobs   = getConnectivity(D)

 
    rThresh= 0.4; % [0..1] A threshold on the correlation.

    [nSamples, nChannels, nHb]=size(D);

    C = nan(nChannels, nChannels, nHb); %Matrix of channel pairwise correlations;

    %This part of the algorithm is HIGHLY inefficient but it does the job for now
    %but might not be sufficiently fast for "real time" neurofeedback

    for iHb = 1:nHb

        for iCh=1:nChannels

            for jCh=iCh:nChannels

                if iCh == jCh

                 C(iCh,jCh,iHb) = 1;

               else

                 C(iCh,jCh,iHb) = corr(D(:,iCh,iHb),D(:,jCh,iHb));

                end
            end

        end

    end

    %Threshold/Binarize C

    tmp = C > rThresh;

    %Finally "merge" accross Hb species

    Aobs = all(tmp,3); %Apply the AND function across Hb species.

== matlab function Neurofeedback_GetConnectivity_IncrementalAvg/getConnectivity3 ==
  data: D input; Aobs output
function Aobs   = getConnectivity(D)

 
    rThresh= 0.6; % [0..1] A threshold on the correlation.

    [nSamples, nChannels, nHb]=size(D);

    C = nan(nChannels, nChannels, nHb); %Matrix of channel pairwise correlations;

    %This part of the algorithm is HIGHLY inefficient but it does the job for now
    %but might not be sufficiently fast for "real time" neurofeedback

    for iHb = 1:nHb
        
        for iCh=1:nChannels
            
            for jCh=iCh:nChannels

                if iCh == jCh

                 C(iCh,jCh,iHb) = 1;

               else

                 C(iCh,jCh,iHb) = 0; %corr(D(:,iCh,iHb),D(:,jCh,iHb));

                end
            end

        end

    end

    %Threshold/Binarize C

    tmp = C > rThresh;

    %Finally "merge" accross Hb species

    Aobs = all(tmp,3); %Apply the AND function across Hb species.

== matlab function Neurofeedback_GetConnectivity_IncrementalAvg/MATLAB Function ==
  data: r input; newAvg output uint16; Qk input uint16; k input
function newAvg = incrementalAverage(r,Qk,k)
%Computes incremental average
%
% newAvg = incrementalAverage(r,Qk,k)
%
%% Computation of the Incremental average
%
%   Let Q_k denote the average of its first k rewards.
%Given this average and a (k+1)-st reward, r_{k+1},
%the average of all $k+1$ rewards can be computed by: 
%
%                 1
%Q_{k+1} = Q_k + --- (r_{k+1}-Q_k)
%                k+1
%
%% Parameters
%
% r - new (k+1)-st reward
% Qk - Current average of the first k rewards
% k - Current number of rewards
%
%% Output
%
% newAvg - The average of all k+1 rewards, Q_{k+1}
%
%
%
%
% Copyright 2010
% @date: 29-Nov-2010
% @author Felipe Orihuela-Espina
% @modified: 29-Nov-2010
%
% See also 
%

newAvg = Qk + (1/(k+1))*(r-Qk);

== matlab function Neurofeedback_GetConnectivity_IncrementalAvg/Subsystem/Hemodynamics1/Efp ==
  data: fjin input; Efp output
function Efp= fcn(fjin)

Efp = (1 - (1 - 0.32).^ (1 ./ fjin))/0.32;

== matlab function Neurofeedback_GetConnectivity_IncrementalAvg/Plant/Human Agent/Hemodynamics/Efp ==
  data: fjin input; Efp output
function Efp= fcn(fjin)

Efp = (1 - (1 - 0.32).^ (1 ./ fjin))/0.32;

== matlab function Neurofeedback_GetConnectivity_IncrementalAvg/Subsystem/Hemodynamics1/Rate Blood Volume/Fv_s ==
  data: Vj input; Vj_expphi output
function Vj_expphi = fcn(Vj)
phi = 0.32;
Vj_expphi = Vj.^(1/phi);

== matlab function Neurofeedback_GetConnectivity_IncrementalAvg/Subsystem/Hemodynamics1/Rate Blood Volume/Vj//Tjv ==
  data: Vj input; Vj_Tjv output
function Vj_Tjv = fcn(Vj)
    Tjv = 2*exp([0;1]);
    Tj = 2*exp([0;0.05]);
Vj_Tjv =(Tj.*Tjv.*Vj);

== matlab function Neurofeedback_GetConnectivity_IncrementalAvg/Subsystem/Neurodynamics1/Jt ==
  data: Zt input; U input; Jt output
function Jt = fcn(Zt, U)
   A = [-0.16 -0.49;-0.02 -0.33];
   nRegions  = size(A,1);
   M = size(U,1); %nStimuli
   simulationLength = size(U,2);
   B = zeros(2,2,2);
   B1 = [0 0; 0 0]; %There must be a B per stimulus
   B2 = [-0.02 -0.77; 0.33 -1.31];
   B(:,:,1) = B1;
   B(:,:,2) = B2;
      assert(M == size(B,3),...
       'Unexpected number of induced connectivity parameters B.');
   T = zeros(nRegions); %nRegions x nRegions
    for t = 1:simulationLength
           for uu = 1:M % Sum (Uj * Bj)
               tmp = U(uu,t)*B(:,:,uu);
               T = -0.5*exp(T + tmp);  
           end
    end
    SI = diag(A);
    A =  A - diag(exp(SI) + (SI));
Jt = (A*Zt) + (T*Zt);
